simulink model "project4V2_storey"  (R2014a)
settings: Solver=FixedStepDiscrete  StartTime=0.0  StopTime=30  FixedStep=5E-5  RelTol=1e-3
undefined symbols (not defined in the file or in its folder): sigbuilder_block
libraries: slrtlib x6, xpcnilib x4, powerlib_meascontrol x2, simulink x1
settings Model: SimulationMode=external  BufferReuse=off  Creator=Jed  LastModifiedBy=Jed
settings SolverCC: EnableConcurrentExecution=on
settings DataIOCC: LimitDataPoints=off
settings OptimizationCC: BlockReduction=off  OptimizeBlockIOStorage=off  BufferReuse=off  GlobalBufferReuse=off  ExpressionFolding=off  LocalBlockOutputs=off
settings HardwareCC: ProdIntDivRoundTo=Zero  ProdEndianess=LittleEndian  ProdHWDeviceType=Generic->32-bit x86 compatible
settings RTWCC: SystemTargetFile=slrt.tlc  TemplateMakefile=slrt_default_tmf  Description=Simulink Real-Time  ProcessScript=slrt_make_rtw_hook  RTWCompilerOptimization=On
settings SimulinkRealTimeCC: GeneratePreprocessorConditionals=Disable all  EnableShiftOperators=on

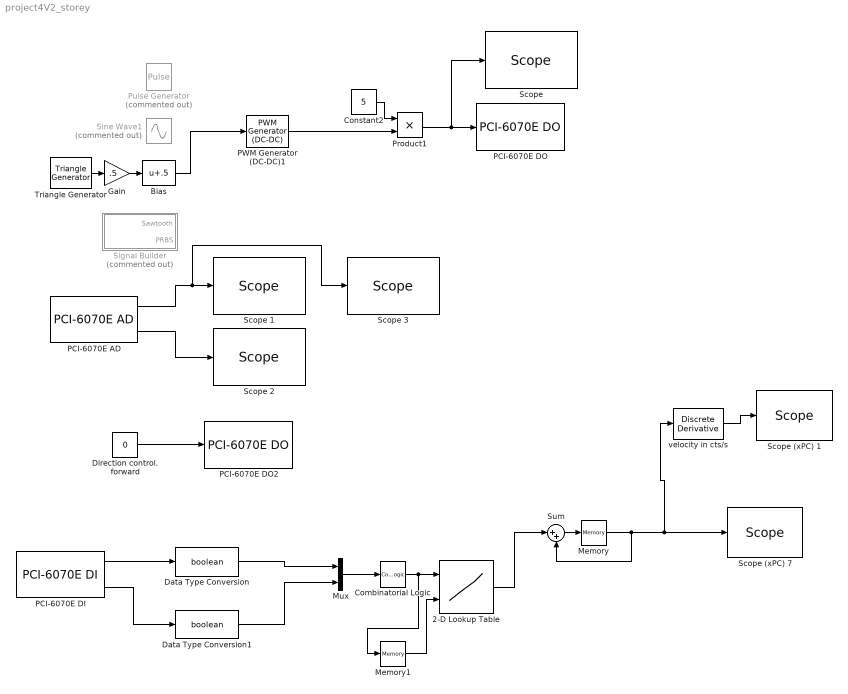
== system project4V2_storey ==
  2-D Lookup Table : Lookup_n-D  BreakpointsForDimension1=[1,2,3,4]  BreakpointsForDimension2=[1,2,3,4]  Table=reshape([0,-1,0,1,1,0,-1,0,0,1,0,-1,-1,0,1,0],4,4)  RndMeth=Simplest  InputSameDT=on
  Bias : Bias  Bias=.5
  Combinatorial Logic : CombinatorialLogic  TruthTable=[1;2;4;3]
  Constant2 : Constant  Value=5  VectorParams1D=off
  Data Type Conversion : DataTypeConversion  OutDataTypeStr=boolean
  Data Type Conversion1 : DataTypeConversion  OutDataTypeStr=boolean
  Direction control. forward : Constant  Value=0  VectorParams1D=off
  Gain : Gain  Gain=.5
  Memory : Memory
  Memory1 : Memory
  Mux : Mux  Inputs=2
  PCI-6070E AD : xpcnilib/A//D/E Series/PCI-6070E AD  channel=[2,1]  range=[-5,-10]  coupling=[2,2]  sampletime=5E-5  slot=[5,0]
  PCI-6070E DI : xpcnilib/Digital Input/E Series/PCI-6070E DI  channel=[2,7]  sampletime=5E-5  slot=[5,0]
  PCI-6070E DO : xpcnilib/Digital Output/E Series/PCI-6070E DO  channel=[1]  reset=[1]  initValue=[0]  sampletime=-1  slot=[5,0]
  PCI-6070E DO2 : xpcnilib/Digital Output/E Series/PCI-6070E DO  channel=[6]  reset=[1]  initValue=[0]  sampletime=-1  slot=[5,0]
  PWM Generator (DC-DC)1 : powerlib_meascontrol/Pulse & Signal Generators/PWM Generator (DC-DC)  Fsw=1011  Ts=5E-5
  Product1 : Product
  Pulse Generator : DiscretePulseGenerator  Commented=on  Period=10000  PulseWidth=4000  PhaseDelay=5000  SampleTime=5E-5
  "Scope " : slrtlib/Displays and Logging/Scope   scopeno=3  scopetype=Host  autostart=on  viewmode=Graphical redraw  formatstr='%15.6f'  grid=on  ylimits=[0,0]  nosamples=6E5  noprepostsamples=0  interleave=1  triggermode=FreeRun  triggersignal=1  trigsignalfromport=off  triggerlevel=0.0  triggerslope=Either  triggerscope=1  triggersample=0  filename=data.dat  mode=Lazy  writesize=512  autorestart=off  dynamicfilemode=off  maxwritefilesize=512*1024^2
  Scope (xPC) 1 : slrtlib/Displays and Logging/Scope   scopeno=5  scopetype=Host  autostart=on  viewmode=Graphical redraw  formatstr='%15.6f'  grid=on  ylimits=[0,0]  nosamples=6E5  noprepostsamples=0  interleave=1  triggermode=FreeRun  triggersignal=1  trigsignalfromport=off  triggerlevel=0.0  triggerslope=Either  triggerscope=1  triggersample=0  filename=data.dat  mode=Lazy  writesize=512  autorestart=off  dynamicfilemode=off  maxwritefilesize=512*1024^2
  Scope (xPC) 7 : slrtlib/Displays and Logging/Scope   scopeno=4  scopetype=Host  autostart=on  viewmode=Graphical redraw  formatstr='%15.6f'  grid=on  ylimits=[0,0]  nosamples=6E5  noprepostsamples=0  interleave=1  triggermode=FreeRun  triggersignal=1  trigsignalfromport=off  triggerlevel=0.0  triggerslope=Either  triggerscope=1  triggersample=0  filename=data.dat  mode=Lazy  writesize=512  autorestart=off  dynamicfilemode=off  maxwritefilesize=512*1024^2
  Scope 1 : slrtlib/Displays and Logging/Scope   scopeno=1  scopetype=Host  autostart=on  viewmode=Graphical redraw  formatstr='%15.6f'  grid=on  ylimits=[0,0]  nosamples=6E5  noprepostsamples=0  interleave=1  triggermode=FreeRun  triggersignal=1  trigsignalfromport=off  triggerlevel=0.0  triggerslope=Either  triggerscope=1  triggersample=0  filename=data.dat  mode=Lazy  writesize=512  autorestart=off  dynamicfilemode=off  maxwritefilesize=512*1024^2
  Scope 2 : slrtlib/Displays and Logging/Scope   scopeno=2  scopetype=Host  autostart=on  viewmode=Graphical redraw  formatstr='%15.6f'  grid=on  ylimits=[0,0]  nosamples=6E5  noprepostsamples=0  interleave=1  triggermode=FreeRun  triggersignal=1  trigsignalfromport=off  triggerlevel=0.0  triggerslope=Either  triggerscope=1  triggersample=0  filename=data.dat  mode=Lazy  writesize=512  autorestart=off  dynamicfilemode=off  maxwritefilesize=512*1024^2
  Scope 3 : slrtlib/Displays and Logging/Scope   scopeno=6  scopetype=Target  autostart=on  viewmode=Graphical redraw  formatstr='%15.6f'  grid=on  ylimits=[0,0]  nosamples=6E5  noprepostsamples=0  interleave=1  triggermode=FreeRun  triggersignal=1  trigsignalfromport=off  triggerlevel=0.0  triggerslope=Either  triggerscope=1  triggersample=0  filename=data.dat  mode=Lazy  writesize=512  autorestart=off  dynamicfilemode=off  maxwritefilesize=512*1024^2
  Signal Builder : Subsystem  Tag=STV Subsys  Commented=on  LoadFcn=sigbuilder_block('load');  StartFcn=sigbuilder_block('start');  StopFcn=sigbuilder_block('stop');  ClipboardFcn=sigbuilder_block('clipboard');  mask(Sigbuilder block){}
      mask help: Simulink:masks:SigbuilderBlock_MD
      mask init:
      | if ~strcmp(get_param(bdroot(gcbh),'SimulationStatus'),'stopped') tuvar = sigbuilder_block('maskInit'); end
      settings: CopyFcn=sigbuilder_block('copy');  DeleteFcn=sigbuilder_block('delete');  ModelCloseFcn=sigbuilder_block('modelClose');  PreSaveFcn=sigbuilder_block('preSave');  PauseFcn=sigbuilder_block('pause');  ContinueFcn=sigbuilder_block('continue');  NameChangeFcn=sigbuilder_block('namechange');  OpenFcn=sigbuilder_block('open',[128.25 255 551.25 399.75 ]);  CloseFcn=sigbuilder_block('close');
      mask Display: plot(0, 0, 100, 100,[2, 2, 32, 32, 2], [68, 8, 8, 68, 68],[32, 2], [38, 38], [32, 19, 2],[53, 60, 44], [32, 17, 17, 2],[16, 16, 31, 31]);txt = getActiveGroup(gcbh);text(2, 100, txt,'verticalAlignment', 'top');
  Sine Wave1 : Sin  Commented=on  Amplitude=0.5  Bias=0.5  Frequency=0.5*(2*3.14159)  SampleTime=0
  Sum : Sum  Inputs=|++  AccumDataTypeStr=int32  OutDataTypeStr=int32
  Triangle Generator : powerlib_meascontrol/Pulse & Signal Generators/Triangle Generator  Freq=3  Phase=0  Ts=5E-5
  velocity in cts/s : simulink/Discrete/Discrete Derivative  gainval=1.0  ICPrevScaledInput=0.0  InputProcessing=Inherited  OutMin=[]  OutMax=[]  OutDataType=fixdt(1, 16)  OutScaling=2^-10  DoSatur=off
  wires:
  Gain/1 -> Bias/1
  PWM Generator (DC-DC)1/1 -> Product1/2
  Constant2/1 -> Product1/1
  Product1/1 -> "Scope "/1, PCI-6070E DO/1
  Bias/1 -> PWM Generator (DC-DC)1/1
  PCI-6070E AD/1 -> Scope 3/1, Scope 1/1
  PCI-6070E AD/2 -> Scope 2/1
  Sum/1 -> Memory/1
  Mux/1 -> Combinatorial Logic/1
  2-D Lookup Table/1 -> Sum/1
  Memory1/1 -> 2-D Lookup Table/2
  Combinatorial Logic/1 -> 2-D Lookup Table/1, Memory1/1
  PCI-6070E DI/1 -> Data Type Conversion/1
  Data Type Conversion/1 -> Mux/1
  PCI-6070E DI/2 -> Data Type Conversion1/1
  Data Type Conversion1/1 -> Mux/2
  velocity in cts/s/1 -> Scope (xPC) 1/1
  Triangle Generator/1 -> Gain/1
  Memory/1 -> Scope (xPC) 7/1, velocity in cts/s/1, Sum/2
  Direction control. forward/1 -> PCI-6070E DO2/1

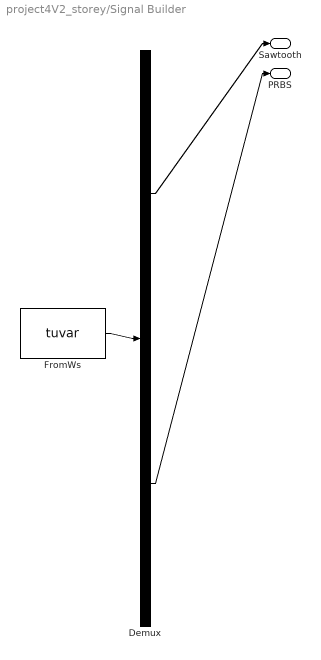
== system project4V2_storey/Signal Builder ==
  Demux : Demux  Tag=STV Demux  Outputs=2
  FromWs : FromWorkspace  Tag=STV FromWs  VariableName=tuvar  SampleTime=0  OutputAfterFinalValue=Setting to zero
      SigBuilderData=|
      | common.afterFinalStr = 'Set to zero'
      | common.sampleTime = '0'
      | dataSet.timeRange = [0 30]
      | dataSet.name = 'Group2'
      | sbobj.Groups.Name = 'Group2'
      | sbobj.Groups.Signals(1).Name = 'Sawtooth'
      | sbobj.Groups.Signals(1).XData = [0 1 1 2 2 3 3 4 4 5 5 6 6 7 7 8 8 9 9 10 30]
      | sbobj.Groups.Signals(1).YData = [0 1 0 1 0 1 0 1 0 1 0 1 0 1 0 1 0 1 0 1 1]
      | sbobj.Groups.Signals(2).Name = 'PRBS'
      | sbobj.Groups.Signals(2).XData = [0 0.133333333333 0.133333333333 0.2 0.2 0.466666666667 0.466666666667 0.533333333333 0.533333333333 0.666666666667 0.666666666667 1 ... (447 elements, 1x447)]
      | sbobj.Groups.Signals(2).YData = [0 0 1 1 0 0 1 1 0 0 1 1 0 0 1 1 0 0 1 1 0 0 1 1 0 0 1 1 0 0 1 1 0 0 1 1 0 0 1 1 0 0 1 1 0 0 1 1 0 0 1 1 0 0 1 1 0 0 1 1 0 0 1 1 0 0 1 1 0 0 1 1 0 0 1 1 0 0 1 1 0 0 1 1 0 0 1 1 0 0 1 1 0 0 1 1 0 0 1 1 0 0 1 1 0 0 1 1 0 0 1 1 0 0 1 1 0 0 1 1 0 0 1 1 0 0 1 1 0 0 1 1 0 0 1 1 0 0 1 1 0 0 1 1 0 0 1 1 0 0 1 1 0 0 1 1 0 0 1 1 0 0 1 1 0 0 1 1 0 0 1 1 0 0 1 1 0 0 1 1 0 0 1 1 0 0 1 1 0 0 1 1 0 0 1 1 0 0 1 1 0 0 1 1 0 0 1 1 0 0 1 1 0 0 1 1 0 0 1 1 0 0 1 1 0 0 1 1 0 0 1 1 0 0 1 1 0 0 1 1 0 0 1 1 0 0 1 1 0 0 1 1 0 0 1 1 0 0 1 1 0 0 1 1 0 0 1 1 0 0 1 1 0 0 1 1 0 0 1 1 0 0 1 1 0 0 1 1 0 0 1 1 0 0 1 1 0 0 1 1 0 0 1 1 0 0 1 1 0 0 1 1 0 0 1 1 0 0 1 1 0 0 1 1 0 0 1 1 0 0 1 1 0 0 1 1 0 0 1 1 0 0 1 1 0 0 1 1 0 0 1 1 0 0 1 1 0 0 1 1 0 0 1 1 0 0 1 1 0 0 1 1 0 0 1 1 0 0 1 1 0 0 1 1 0 0 1 1 0 0 1 1 0 0 1 1 0 0 1 1 0 0 1 1 0 0 1 1 0 0 1 1 0 0 1 1 0 0 1 1 0 0 1 1 0 0 1 1 0 0 1 1 0 0 1 1 0 0 1 1 0 0 1 1 0 0 1]
      | sbobj.Groups.TimeRange = [0 30]
  Sawtooth : Outport  Tag=STV Outport
  PRBS : Outport  Tag=STV Outport  Port=2
  wires:
  FromWs/1 -> Demux/1
  Demux/1 -> Sawtooth/1
  Demux/2 -> PRBS/1
